simulink model "Week1problem4"  (R2020b)
settings: Solver=VariableStepAuto  StartTime=0.0  StopTime=10.0  RelTol=1e-3
settings Model: Creator=Admin  LastModifiedBy=Admin

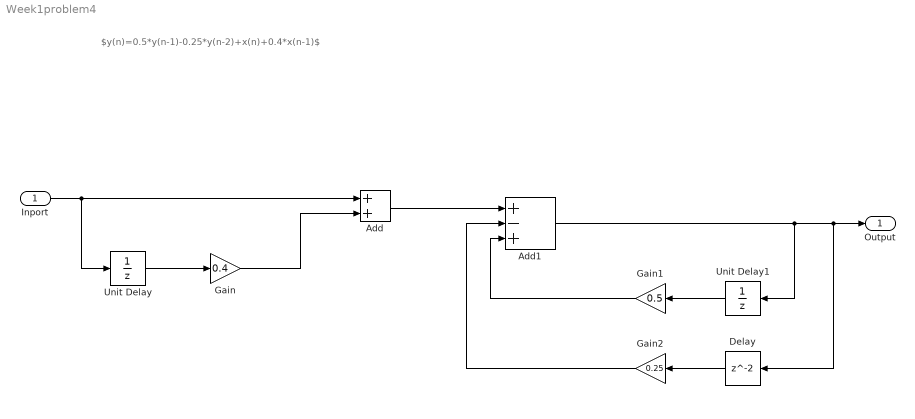
== system Week1problem4 ==
  note: $y(n)=0.5*y(n-1)-0.25*y(n-2)+x(n)+0.4*x(n-1)$
  Inport : Inport
  Add : Sum
  Add1 : Sum  Inputs=+-+
  Delay : Delay
  Gain : Gain  Gain=0.4
  Gain1 : Gain  Gain=0.5
  Gain2 : Gain  Gain=0.25
  Unit Delay : UnitDelay  SampleTime=-1  HasFrameUpgradeWarning=on
  Unit Delay1 : UnitDelay  SampleTime=-1  HasFrameUpgradeWarning=on
  Output : Outport
  wires:
  Inport/1 -> Unit Delay/1, Add/1
  Unit Delay/1 -> Gain/1
  Gain/1 -> Add/2
  Add/1 -> Add1/1
  Gain1/1 -> Add1/3
  Add1/1 -> Unit Delay1/1, Delay/1, Output/1
  Unit Delay1/1 -> Gain1/1
  Delay/1 -> Gain2/1
  Gain2/1 -> Add1/2
